simulink model "MotorSample"  (R2026a)
settings: Solver=VariableStepAuto
libraries: robotcorelib x1
settings Model: Creator=eqtran103  LastModifiedBy=eqtran103

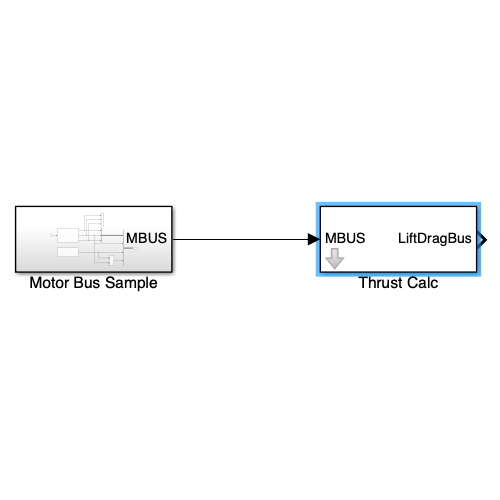
[thumbnail: Simulink's stored preview of the top-level diagram]
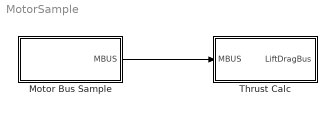
== system MotorSample ==
  Motor Bus Sample : Subsystem
  Thrust Calc : Subsystem  mask{L_C=1, L_to_D=1}
      mask prompts: L_C "Lift Coefficent (N/(rad/s)^2)"; L_to_D "Lift to Drag (m)"
  wires:
  Motor Bus Sample/1(MBUS) -> Thrust Calc/1(MBUS)

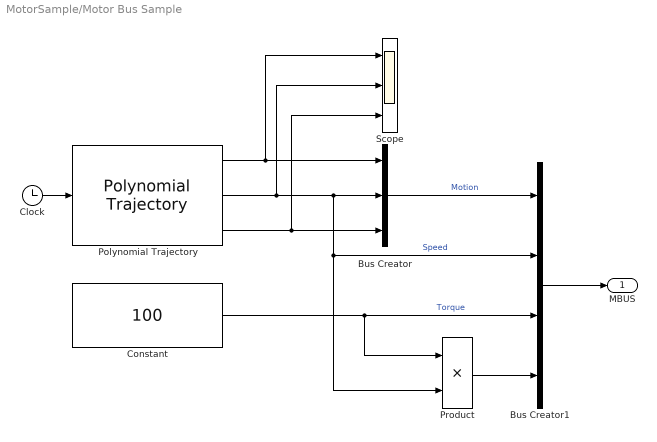
== system MotorSample/Motor Bus Sample ==
  Bus Creator : BusCreator  Inputs=3
  Bus Creator1 : BusCreator  Inputs=4
  Clock : Clock
  Constant : Constant  Value=100
  Polynomial Trajectory : robotcorelib/Polynomial Trajectory  WaypointSource=Internal  Waypoints=[0,-10000]  TimePoints=[1,6]  TimeInterval=[ 1, 4 ]  Method=Cubic Polynomial  ParameterSource=Internal  VelocityBoundaryCondition=zeros(1, 2 )  AccelerationBoundaryCondition=zeros( 1, 2 )  SimulateUsing=Interpreted execution
  Product : Product
  Scope : Scope  NumInputPorts=3
      settings: ActiveDisplayYMinimum=-11250  ActiveDisplayYMaximum=1249.9999999999998
  MBUS : Outport
  wires:
  Polynomial Trajectory/3 -> Scope/3, Bus Creator/3
  Polynomial Trajectory/2 -> Scope/2, Bus Creator1/2, Product/2, Bus Creator/2  "Speed"
  Polynomial Trajectory/1 -> Scope/1, Bus Creator/1
  Bus Creator/1 -> Bus Creator1/1  "Motion"
  Constant/1 -> Product/1, Bus Creator1/3  "Torque"
  Product/1 -> Bus Creator1/4
  Bus Creator1/1 -> MBUS/1
  Clock/1 -> Polynomial Trajectory/1

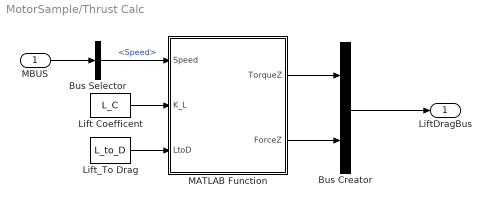
== system MotorSample/Thrust Calc ==
  MBUS : Inport
  Bus Creator : BusCreator  Inputs=2
  Bus Selector : BusSelector  OutputSignals=Speed
  Lift Coefficent : Constant  Value=L_C
  Lift_To Drag : Constant  Value=L_to_D
  MATLAB Function : MATLAB Function  TreatAsAtomicUnit=on
  LiftDragBus : Outport
  wires:
  MBUS/1 -> Bus Selector/1
  Bus Selector/1 -> MATLAB Function/1(Speed)  "<Speed>"
  MATLAB Function/1(TorqueZ) -> Bus Creator/1
  MATLAB Function/2(ForceZ) -> Bus Creator/2
  Bus Creator/1 -> LiftDragBus/1
  Lift Coefficent/1 -> MATLAB Function/2(K_L)
  Lift_To Drag/1 -> MATLAB Function/3(LtoD)

== matlab function MotorSample/Thrust Calc/MATLAB Function ==
  data: Speed input; TorqueZ output; K_L input; LtoD input; ForceZ output
function [TorqueZ,ForceZ] = fcn(Speed, K_L, LtoD)
% Speed - propeller rotational speed (signed)
% K_L   - lift coefficient gain (speed^2 -> thrust)
% LtoD  - lift-to-drag ratio (thrust -> load torque)
% Torque - resulting load torque on the motor
ForceZ = K_L * Speed^2;
TorqueZ = K_L * Speed^2 * sign(Speed) / LtoD;
end
